simulink model "w2_warplab_trigger_proc"  (Simulink 7.7)
settings: Solver=ode45  StartTime=0.0  StopTime=1000  RelTol=1e-3
InitFcn:
  | w2_warplab_trigger_proc_init
StartFcn:
  | w2_warplab_trigger_proc_init
undefined symbols (not defined in the file or in its folder): gcbh, xlBlockLoadCallback, xlGetNormalizedPeriod
libraries: xbsIndex_r4 x819, simulink x1
(part 6 of 6)

== system w2_warplab_trigger_proc/Trigger Sources/Energy/AntB Detector/Busy Detection ==
  Avg RSSI : Inport
  Reset : Inport  Port=2
  en : Inport  Port=3
  Convert1 : xbsIndex_r4/Convert  gui_display_data_type=Fixed-point  arith_type=Unsigned  n_bits=1  bin_pt=0  float_type=Single  exp_bits=8  fraction_bits=24  quantization=Truncate  overflow=Wrap  en=off  latency=0  dbl_ovrd=off  pipeline=off  block_type=convert
      settings: block_version=VER_STRING_GOES_HERE
  Counter1 : xbsIndex_r4/Counter  cnt_type=Free Running  cnt_to=Inf  operation=Up  start_count=0  cnt_by_val=1  arith_type=Unsigned  n_bits=11  bin_pt=0  load_pin=off  rst=on  en=on  explicit_period=off  period=4  dbl_ovrd=off  use_behavioral_HDL=off  implementation=Fabric  use_rpm=off  block_type=counter
  Inverter1 : xbsIndex_r4/Inverter  en=off  latency=0  dbl_ovrd=off  block_type=inv
      settings: xl_area=[0 0 0 0 0 0 0]  block_version=8.2
  Logical : xbsIndex_r4/Logical  logical_function=AND  inputs=2  en=off  latency=0  precision=Full  arith_type=Unsigned  n_bits=16  bin_pt=0  align_bp=on  dbl_ovrd=off  block_type=logical
  Logical1 : xbsIndex_r4/Logical  logical_function=OR  inputs=2  en=off  latency=0  precision=Full  arith_type=Unsigned  n_bits=16  bin_pt=0  align_bp=on  dbl_ovrd=off  block_type=logical
  Relational2 : xbsIndex_r4/Relational  mode=a>b  en=off  latency=0  dbl_ovrd=off  block_type=relational
      settings: block_version=VER_STRING_GOES_HERE
  Relational3 : xbsIndex_r4/Relational  mode=a>b  en=off  latency=0  dbl_ovrd=off  block_type=relational
      settings: block_version=VER_STRING_GOES_HERE
  S-R Latch : Subsystem
  Busy : Outport
  wires:
  [pktDet_energyThresh_busy] -> Relational2/2
  Reset/1 -> Logical1/1
  Logical1/1 -> Counter1/1, S-R Latch/1(R)
  Inverter1/1 -> Logical1/2
  Counter1/1 -> Relational3/1
  [pktDet_duration_busy] -> Relational3/2
  Relational3/1 -> S-R Latch/2(S)
  S-R Latch/1(Q) -> Convert1/1
  Avg RSSI/1 -> Relational2/1
  Convert1/1 -> Busy/1
  Logical/1 -> Counter1/2
  Relational2/1 -> Logical/1, Inverter1/1
  en/1 -> Logical/2

== system w2_warplab_trigger_proc/Trigger Sources/Energy/AntB Detector/Idle Detection ==
  Avg RSSI : Inport
  Reset : Inport  Port=2
  en : Inport  Port=3
  Convert1 : xbsIndex_r4/Convert  gui_display_data_type=Fixed-point  arith_type=Unsigned  n_bits=1  bin_pt=0  float_type=Single  exp_bits=8  fraction_bits=24  quantization=Truncate  overflow=Wrap  en=off  latency=0  dbl_ovrd=off  pipeline=off  block_type=convert
      settings: block_version=VER_STRING_GOES_HERE
  Counter1 : xbsIndex_r4/Counter  cnt_type=Free Running  cnt_to=Inf  operation=Up  start_count=0  cnt_by_val=1  arith_type=Unsigned  n_bits=11  bin_pt=0  load_pin=off  rst=on  en=on  explicit_period=off  period=4  dbl_ovrd=off  use_behavioral_HDL=off  implementation=Fabric  use_rpm=off  block_type=counter
  Inverter1 : xbsIndex_r4/Inverter  en=off  latency=0  dbl_ovrd=off  block_type=inv
      settings: xl_area=[0 0 0 0 0 0 0]  block_version=8.2
  Logical : xbsIndex_r4/Logical  logical_function=AND  inputs=2  en=off  latency=0  precision=Full  arith_type=Unsigned  n_bits=16  bin_pt=0  align_bp=on  dbl_ovrd=off  block_type=logical
  Logical1 : xbsIndex_r4/Logical  logical_function=OR  inputs=2  en=off  latency=0  precision=Full  arith_type=Unsigned  n_bits=16  bin_pt=0  align_bp=on  dbl_ovrd=off  block_type=logical
  Relational2 : xbsIndex_r4/Relational  mode=a<b  en=off  latency=0  dbl_ovrd=off  block_type=relational
      settings: block_version=VER_STRING_GOES_HERE
  Relational3 : xbsIndex_r4/Relational  mode=a>b  en=off  latency=0  dbl_ovrd=off  block_type=relational
      settings: block_version=VER_STRING_GOES_HERE
  S-R Latch : Subsystem
  Idle : Outport
  wires:
  Convert1/1 -> Idle/1
  Avg RSSI/1 -> Relational2/1
  S-R Latch/1(Q) -> Convert1/1
  Relational3/1 -> S-R Latch/2(S)
  [pktDet_duration_idle] -> Relational3/2
  Counter1/1 -> Relational3/1
  Inverter1/1 -> Logical1/2
  Logical1/1 -> Counter1/1, S-R Latch/1(R)
  Reset/1 -> Logical1/1
  Relational2/1 -> Logical/1, Inverter1/1
  [pktDet_energyThresh_idle] -> Relational2/2
  en/1 -> Logical/2
  Logical/1 -> Counter1/2

== system w2_warplab_trigger_proc/Trigger Sources/Energy/AntB Detector/Running Sum ==
  note: This block impelemnts a variable-length running sum.
      | For a sum y(n) of the previous N samples of sequence x(n), it implements
      | y(n) = y(n-1) + x(n) - x(n-N)
      | This requires a careful reset procedure, where the full shift register
      | is zerored out. Otherwise the feedback-based sum stops working.
  RSSI : Inport
  reset : Inport  Port=2
  avglen : Inport  Port=3
  en : Inport  Port=4
  ASR : xbsIndex_r4/Addressable Shift Register  infer_latency=on  depth=2  initVector=[0]  en=on  dbl_ovrd=off  use_behavioral_HDL=off  Optimization=Resource  use_rpm=off  block_type=addrsr
      settings: infoedit="Delay of configurable length.  Any element in the delay line can be addressed and driven onto the output port.<br><br>Hardware notes: This block is implemented using SRL16s. If Virtex-4 or Spartan-3 device is used, multiple SRLC16s are cascaded together."  block_version=VER_STRING_GOES_HERE
  Accumulator : xbsIndex_r4/Accumulator  operation=Add  n_bits=17  overflow=Flag as error  scale=1  rst=on  infoeditControl=reset for floating point data type must be asserted for a minimum of 2 cycles  hasbypass=off  en=on  latency=0  dbl_ovrd=off  msb_inp=100  msb=100  lsb=-100  use_behavioral_HDL=on  implementation=Fabric  block_type=accum
      settings: block_version=VER_STRING_GOES_HERE
  AddSub : xbsIndex_r4/AddSub  mode=Subtraction  use_carryin=off  use_carryout=off  en=off  latency=0  precision=Full  arith_type=Unsigned  n_bits=10  bin_pt=0  quantization=Truncate  overflow=Wrap  dbl_ovrd=off  use_behavioral_HDL=off  hw_selection=Fabric  pipelined=off  use_rpm=on  block_type=addsub
      settings: block_version=VER_STRING_GOES_HERE
  Convert7 : xbsIndex_r4/Convert  gui_display_data_type=Fixed-point  arith_type=Unsigned  n_bits=17  bin_pt=0  float_type=Single  exp_bits=8  fraction_bits=24  quantization=Truncate  overflow=Saturate  en=off  latency=0  dbl_ovrd=off  pipeline=off  block_type=convert
      settings: block_version=10.1.3
  Logical : xbsIndex_r4/Logical  logical_function=OR  inputs=2  en=off  latency=0  precision=Full  arith_type=Unsigned  n_bits=16  bin_pt=0  align_bp=on  dbl_ovrd=off  block_type=logical
  Long Reset Gen : Subsystem
  Register : xbsIndex_r4/Register  init=0  rst=on  en=off  dbl_ovrd=off  block_type=register
      settings: block_version=VER_STRING_GOES_HERE
  avg : Outport
  wires:
  en/1 -> Accumulator/3, ASR/3
  Convert7/1 -> avg/1
  Long Reset Gen/1(reset_out) -> Logical/1
  reset/1 -> Logical/2, Long Reset Gen/2(reset_in)
  Logical/1 -> Accumulator/2, Register/2
  Accumulator/1 -> Convert7/1
  RSSI/1 -> Register/1
  avglen/1 -> Long Reset Gen/1(duration), ASR/2
  Register/1 -> AddSub/1, ASR/1
  AddSub/1 -> Accumulator/1
  ASR/1 -> AddSub/2

== system w2_warplab_trigger_proc/Trigger Sources/Energy/AntC Detector/Busy Detection ==
  Avg RSSI : Inport
  Reset : Inport  Port=2
  en : Inport  Port=3
  Convert1 : xbsIndex_r4/Convert  gui_display_data_type=Fixed-point  arith_type=Unsigned  n_bits=1  bin_pt=0  float_type=Single  exp_bits=8  fraction_bits=24  quantization=Truncate  overflow=Wrap  en=off  latency=0  dbl_ovrd=off  pipeline=off  block_type=convert
      settings: block_version=VER_STRING_GOES_HERE
  Counter1 : xbsIndex_r4/Counter  cnt_type=Free Running  cnt_to=Inf  operation=Up  start_count=0  cnt_by_val=1  arith_type=Unsigned  n_bits=11  bin_pt=0  load_pin=off  rst=on  en=on  explicit_period=off  period=4  dbl_ovrd=off  use_behavioral_HDL=off  implementation=Fabric  use_rpm=off  block_type=counter
  Inverter1 : xbsIndex_r4/Inverter  en=off  latency=0  dbl_ovrd=off  block_type=inv
      settings: xl_area=[0 0 0 0 0 0 0]  block_version=8.2
  Logical : xbsIndex_r4/Logical  logical_function=AND  inputs=2  en=off  latency=0  precision=Full  arith_type=Unsigned  n_bits=16  bin_pt=0  align_bp=on  dbl_ovrd=off  block_type=logical
  Logical1 : xbsIndex_r4/Logical  logical_function=OR  inputs=2  en=off  latency=0  precision=Full  arith_type=Unsigned  n_bits=16  bin_pt=0  align_bp=on  dbl_ovrd=off  block_type=logical
  Relational2 : xbsIndex_r4/Relational  mode=a>b  en=off  latency=0  dbl_ovrd=off  block_type=relational
      settings: block_version=VER_STRING_GOES_HERE
  Relational3 : xbsIndex_r4/Relational  mode=a>b  en=off  latency=0  dbl_ovrd=off  block_type=relational
      settings: block_version=VER_STRING_GOES_HERE
  S-R Latch : Subsystem
  Busy : Outport
  wires:
  [pktDet_energyThresh_busy] -> Relational2/2
  Reset/1 -> Logical1/1
  Logical1/1 -> Counter1/1, S-R Latch/1(R)
  Inverter1/1 -> Logical1/2
  Counter1/1 -> Relational3/1
  [pktDet_duration_busy] -> Relational3/2
  Relational3/1 -> S-R Latch/2(S)
  S-R Latch/1(Q) -> Convert1/1
  Avg RSSI/1 -> Relational2/1
  Convert1/1 -> Busy/1
  Logical/1 -> Counter1/2
  Relational2/1 -> Logical/1, Inverter1/1
  en/1 -> Logical/2

== system w2_warplab_trigger_proc/Trigger Sources/Energy/AntC Detector/Idle Detection ==
  Avg RSSI : Inport
  Reset : Inport  Port=2
  en : Inport  Port=3
  Convert1 : xbsIndex_r4/Convert  gui_display_data_type=Fixed-point  arith_type=Unsigned  n_bits=1  bin_pt=0  float_type=Single  exp_bits=8  fraction_bits=24  quantization=Truncate  overflow=Wrap  en=off  latency=0  dbl_ovrd=off  pipeline=off  block_type=convert
      settings: block_version=VER_STRING_GOES_HERE
  Counter1 : xbsIndex_r4/Counter  cnt_type=Free Running  cnt_to=Inf  operation=Up  start_count=0  cnt_by_val=1  arith_type=Unsigned  n_bits=11  bin_pt=0  load_pin=off  rst=on  en=on  explicit_period=off  period=4  dbl_ovrd=off  use_behavioral_HDL=off  implementation=Fabric  use_rpm=off  block_type=counter
  Inverter1 : xbsIndex_r4/Inverter  en=off  latency=0  dbl_ovrd=off  block_type=inv
      settings: xl_area=[0 0 0 0 0 0 0]  block_version=8.2
  Logical : xbsIndex_r4/Logical  logical_function=AND  inputs=2  en=off  latency=0  precision=Full  arith_type=Unsigned  n_bits=16  bin_pt=0  align_bp=on  dbl_ovrd=off  block_type=logical
  Logical1 : xbsIndex_r4/Logical  logical_function=OR  inputs=2  en=off  latency=0  precision=Full  arith_type=Unsigned  n_bits=16  bin_pt=0  align_bp=on  dbl_ovrd=off  block_type=logical
  Relational2 : xbsIndex_r4/Relational  mode=a<b  en=off  latency=0  dbl_ovrd=off  block_type=relational
      settings: block_version=VER_STRING_GOES_HERE
  Relational3 : xbsIndex_r4/Relational  mode=a>b  en=off  latency=0  dbl_ovrd=off  block_type=relational
      settings: block_version=VER_STRING_GOES_HERE
  S-R Latch : Subsystem
  Idle : Outport
  wires:
  Convert1/1 -> Idle/1
  Avg RSSI/1 -> Relational2/1
  S-R Latch/1(Q) -> Convert1/1
  Relational3/1 -> S-R Latch/2(S)
  [pktDet_duration_idle] -> Relational3/2
  Counter1/1 -> Relational3/1
  Inverter1/1 -> Logical1/2
  Logical1/1 -> Counter1/1, S-R Latch/1(R)
  Reset/1 -> Logical1/1
  Relational2/1 -> Logical/1, Inverter1/1
  [pktDet_energyThresh_idle] -> Relational2/2
  en/1 -> Logical/2
  Logical/1 -> Counter1/2

== system w2_warplab_trigger_proc/Trigger Sources/Energy/AntC Detector/Running Sum ==
  note: This block impelemnts a variable-length running sum.
      | For a sum y(n) of the previous N samples of sequence x(n), it implements
      | y(n) = y(n-1) + x(n) - x(n-N)
      | This requires a careful reset procedure, where the full shift register
      | is zerored out. Otherwise the feedback-based sum stops working.
  RSSI : Inport
  reset : Inport  Port=2
  avglen : Inport  Port=3
  en : Inport  Port=4
  ASR : xbsIndex_r4/Addressable Shift Register  infer_latency=on  depth=2  initVector=[0]  en=on  dbl_ovrd=off  use_behavioral_HDL=off  Optimization=Resource  use_rpm=off  block_type=addrsr
      settings: infoedit="Delay of configurable length.  Any element in the delay line can be addressed and driven onto the output port.<br><br>Hardware notes: This block is implemented using SRL16s. If Virtex-4 or Spartan-3 device is used, multiple SRLC16s are cascaded together."  block_version=VER_STRING_GOES_HERE
  Accumulator : xbsIndex_r4/Accumulator  operation=Add  n_bits=17  overflow=Flag as error  scale=1  rst=on  infoeditControl=reset for floating point data type must be asserted for a minimum of 2 cycles  hasbypass=off  en=on  latency=0  dbl_ovrd=off  msb_inp=100  msb=100  lsb=-100  use_behavioral_HDL=on  implementation=Fabric  block_type=accum
      settings: block_version=VER_STRING_GOES_HERE
  AddSub : xbsIndex_r4/AddSub  mode=Subtraction  use_carryin=off  use_carryout=off  en=off  latency=0  precision=Full  arith_type=Unsigned  n_bits=10  bin_pt=0  quantization=Truncate  overflow=Wrap  dbl_ovrd=off  use_behavioral_HDL=off  hw_selection=Fabric  pipelined=off  use_rpm=on  block_type=addsub
      settings: block_version=VER_STRING_GOES_HERE
  Convert7 : xbsIndex_r4/Convert  gui_display_data_type=Fixed-point  arith_type=Unsigned  n_bits=17  bin_pt=0  float_type=Single  exp_bits=8  fraction_bits=24  quantization=Truncate  overflow=Saturate  en=off  latency=0  dbl_ovrd=off  pipeline=off  block_type=convert
      settings: block_version=10.1.3
  Logical : xbsIndex_r4/Logical  logical_function=OR  inputs=2  en=off  latency=0  precision=Full  arith_type=Unsigned  n_bits=16  bin_pt=0  align_bp=on  dbl_ovrd=off  block_type=logical
  Long Reset Gen : Subsystem
  Register : xbsIndex_r4/Register  init=0  rst=on  en=off  dbl_ovrd=off  block_type=register
      settings: block_version=VER_STRING_GOES_HERE
  avg : Outport
  wires:
  ASR/1 -> AddSub/2
  AddSub/1 -> Accumulator/1
  Register/1 -> ASR/1, AddSub/1
  avglen/1 -> ASR/2, Long Reset Gen/1(duration)
  RSSI/1 -> Register/1
  Accumulator/1 -> Convert7/1
  Logical/1 -> Register/2, Accumulator/2
  reset/1 -> Long Reset Gen/2(reset_in), Logical/2
  Long Reset Gen/1(reset_out) -> Logical/1
  Convert7/1 -> avg/1
  en/1 -> ASR/3, Accumulator/3

== system w2_warplab_trigger_proc/Trigger Sources/Energy/AntD Detector/Busy Detection ==
  Avg RSSI : Inport
  Reset : Inport  Port=2
  en : Inport  Port=3
  Convert1 : xbsIndex_r4/Convert  gui_display_data_type=Fixed-point  arith_type=Unsigned  n_bits=1  bin_pt=0  float_type=Single  exp_bits=8  fraction_bits=24  quantization=Truncate  overflow=Wrap  en=off  latency=0  dbl_ovrd=off  pipeline=off  block_type=convert
      settings: block_version=VER_STRING_GOES_HERE
  Counter1 : xbsIndex_r4/Counter  cnt_type=Free Running  cnt_to=Inf  operation=Up  start_count=0  cnt_by_val=1  arith_type=Unsigned  n_bits=11  bin_pt=0  load_pin=off  rst=on  en=on  explicit_period=off  period=4  dbl_ovrd=off  use_behavioral_HDL=off  implementation=Fabric  use_rpm=off  block_type=counter
  Inverter1 : xbsIndex_r4/Inverter  en=off  latency=0  dbl_ovrd=off  block_type=inv
      settings: xl_area=[0 0 0 0 0 0 0]  block_version=8.2
  Logical : xbsIndex_r4/Logical  logical_function=AND  inputs=2  en=off  latency=0  precision=Full  arith_type=Unsigned  n_bits=16  bin_pt=0  align_bp=on  dbl_ovrd=off  block_type=logical
  Logical1 : xbsIndex_r4/Logical  logical_function=OR  inputs=2  en=off  latency=0  precision=Full  arith_type=Unsigned  n_bits=16  bin_pt=0  align_bp=on  dbl_ovrd=off  block_type=logical
  Relational2 : xbsIndex_r4/Relational  mode=a>b  en=off  latency=0  dbl_ovrd=off  block_type=relational
      settings: block_version=VER_STRING_GOES_HERE
  Relational3 : xbsIndex_r4/Relational  mode=a>b  en=off  latency=0  dbl_ovrd=off  block_type=relational
      settings: block_version=VER_STRING_GOES_HERE
  S-R Latch : Subsystem
  Busy : Outport
  wires:
  [pktDet_energyThresh_busy] -> Relational2/2
  Reset/1 -> Logical1/1
  Logical1/1 -> Counter1/1, S-R Latch/1(R)
  Inverter1/1 -> Logical1/2
  Counter1/1 -> Relational3/1
  [pktDet_duration_busy] -> Relational3/2
  Relational3/1 -> S-R Latch/2(S)
  S-R Latch/1(Q) -> Convert1/1
  Avg RSSI/1 -> Relational2/1
  Convert1/1 -> Busy/1
  Logical/1 -> Counter1/2
  Relational2/1 -> Logical/1, Inverter1/1
  en/1 -> Logical/2

== system w2_warplab_trigger_proc/Trigger Sources/Energy/AntD Detector/Idle Detection ==
  Avg RSSI : Inport
  Reset : Inport  Port=2
  en : Inport  Port=3
  Convert1 : xbsIndex_r4/Convert  gui_display_data_type=Fixed-point  arith_type=Unsigned  n_bits=1  bin_pt=0  float_type=Single  exp_bits=8  fraction_bits=24  quantization=Truncate  overflow=Wrap  en=off  latency=0  dbl_ovrd=off  pipeline=off  block_type=convert
      settings: block_version=VER_STRING_GOES_HERE
  Counter1 : xbsIndex_r4/Counter  cnt_type=Free Running  cnt_to=Inf  operation=Up  start_count=0  cnt_by_val=1  arith_type=Unsigned  n_bits=11  bin_pt=0  load_pin=off  rst=on  en=on  explicit_period=off  period=4  dbl_ovrd=off  use_behavioral_HDL=off  implementation=Fabric  use_rpm=off  block_type=counter
  Inverter1 : xbsIndex_r4/Inverter  en=off  latency=0  dbl_ovrd=off  block_type=inv
      settings: xl_area=[0 0 0 0 0 0 0]  block_version=8.2
  Logical : xbsIndex_r4/Logical  logical_function=AND  inputs=2  en=off  latency=0  precision=Full  arith_type=Unsigned  n_bits=16  bin_pt=0  align_bp=on  dbl_ovrd=off  block_type=logical
  Logical1 : xbsIndex_r4/Logical  logical_function=OR  inputs=2  en=off  latency=0  precision=Full  arith_type=Unsigned  n_bits=16  bin_pt=0  align_bp=on  dbl_ovrd=off  block_type=logical
  Relational2 : xbsIndex_r4/Relational  mode=a<b  en=off  latency=0  dbl_ovrd=off  block_type=relational
      settings: block_version=VER_STRING_GOES_HERE
  Relational3 : xbsIndex_r4/Relational  mode=a>b  en=off  latency=0  dbl_ovrd=off  block_type=relational
      settings: block_version=VER_STRING_GOES_HERE
  S-R Latch : Subsystem
  Idle : Outport
  wires:
  Convert1/1 -> Idle/1
  Avg RSSI/1 -> Relational2/1
  S-R Latch/1(Q) -> Convert1/1
  Relational3/1 -> S-R Latch/2(S)
  [pktDet_duration_idle] -> Relational3/2
  Counter1/1 -> Relational3/1
  Inverter1/1 -> Logical1/2
  Logical1/1 -> Counter1/1, S-R Latch/1(R)
  Reset/1 -> Logical1/1
  Relational2/1 -> Logical/1, Inverter1/1
  [pktDet_energyThresh_idle] -> Relational2/2
  en/1 -> Logical/2
  Logical/1 -> Counter1/2

== system w2_warplab_trigger_proc/Trigger Sources/Energy/AntD Detector/Running Sum ==
  note: This block impelemnts a variable-length running sum.
      | For a sum y(n) of the previous N samples of sequence x(n), it implements
      | y(n) = y(n-1) + x(n) - x(n-N)
      | This requires a careful reset procedure, where the full shift register
      | is zerored out. Otherwise the feedback-based sum stops working.
  RSSI : Inport
  reset : Inport  Port=2
  avglen : Inport  Port=3
  en : Inport  Port=4
  ASR : xbsIndex_r4/Addressable Shift Register  infer_latency=on  depth=2  initVector=[0]  en=on  dbl_ovrd=off  use_behavioral_HDL=off  Optimization=Resource  use_rpm=off  block_type=addrsr
      settings: infoedit="Delay of configurable length.  Any element in the delay line can be addressed and driven onto the output port.<br><br>Hardware notes: This block is implemented using SRL16s. If Virtex-4 or Spartan-3 device is used, multiple SRLC16s are cascaded together."  block_version=VER_STRING_GOES_HERE
  Accumulator : xbsIndex_r4/Accumulator  operation=Add  n_bits=17  overflow=Flag as error  scale=1  rst=on  infoeditControl=reset for floating point data type must be asserted for a minimum of 2 cycles  hasbypass=off  en=on  latency=0  dbl_ovrd=off  msb_inp=100  msb=100  lsb=-100  use_behavioral_HDL=on  implementation=Fabric  block_type=accum
      settings: block_version=VER_STRING_GOES_HERE
  AddSub : xbsIndex_r4/AddSub  mode=Subtraction  use_carryin=off  use_carryout=off  en=off  latency=0  precision=Full  arith_type=Unsigned  n_bits=10  bin_pt=0  quantization=Truncate  overflow=Wrap  dbl_ovrd=off  use_behavioral_HDL=off  hw_selection=Fabric  pipelined=off  use_rpm=on  block_type=addsub
      settings: block_version=VER_STRING_GOES_HERE
  Convert7 : xbsIndex_r4/Convert  gui_display_data_type=Fixed-point  arith_type=Unsigned  n_bits=17  bin_pt=0  float_type=Single  exp_bits=8  fraction_bits=24  quantization=Truncate  overflow=Saturate  en=off  latency=0  dbl_ovrd=off  pipeline=off  block_type=convert
      settings: block_version=10.1.3
  Logical : xbsIndex_r4/Logical  logical_function=OR  inputs=2  en=off  latency=0  precision=Full  arith_type=Unsigned  n_bits=16  bin_pt=0  align_bp=on  dbl_ovrd=off  block_type=logical
  Long Reset Gen : Subsystem
  Register : xbsIndex_r4/Register  init=0  rst=on  en=off  dbl_ovrd=off  block_type=register
      settings: block_version=VER_STRING_GOES_HERE
  avg : Outport
  wires:
  en/1 -> Accumulator/3, ASR/3
  Convert7/1 -> avg/1
  Long Reset Gen/1(reset_out) -> Logical/1
  reset/1 -> Logical/2, Long Reset Gen/2(reset_in)
  Logical/1 -> Accumulator/2, Register/2
  Accumulator/1 -> Convert7/1
  RSSI/1 -> Register/1
  avglen/1 -> Long Reset Gen/1(duration), ASR/2
  Register/1 -> AddSub/1, ASR/1
  AddSub/1 -> Accumulator/1
  ASR/1 -> AddSub/2

== system w2_warplab_trigger_proc/Trigger Sources/Energy/AntA Detector/Busy Detection/S-R Latch ==
  R : Inport
  S : Inport  Port=2
  Constant1 : xbsIndex_r4/Constant  const=1  gui_display_data_type=Fixed-point  arith_type=Boolean  n_bits=1  bin_pt=0  preci_type=Single  exp_width=8  frac_width=24  explicit_period=off  period=1  equ=P=C  opselect=C  inp2=PCIN>>17  opr=+  inp1=P  carry=CIN  dbl_ovrd=off  block_type=constant
      settings: block_version=VER_STRING_GOES_HERE
  Register2 : xbsIndex_r4/Register  init=0  rst=on  en=on  dbl_ovrd=off  block_type=register
      settings: xl_area=[1 1 0 0 0 0 0]  block_version=VER_STRING_GOES_HERE
  Q : Outport
  wires:
  Constant1/1 -> Register2/1
  R/1 -> Register2/2
  Register2/1 -> Q/1
  S/1 -> Register2/3

== system w2_warplab_trigger_proc/Trigger Sources/Energy/AntA Detector/Idle Detection/S-R Latch ==
  R : Inport
  S : Inport  Port=2
  Constant1 : xbsIndex_r4/Constant  const=1  gui_display_data_type=Fixed-point  arith_type=Boolean  n_bits=1  bin_pt=0  preci_type=Single  exp_width=8  frac_width=24  explicit_period=off  period=1  equ=P=C  opselect=C  inp2=PCIN>>17  opr=+  inp1=P  carry=CIN  dbl_ovrd=off  block_type=constant
      settings: block_version=VER_STRING_GOES_HERE
  Register2 : xbsIndex_r4/Register  init=0  rst=on  en=on  dbl_ovrd=off  block_type=register
      settings: xl_area=[1 1 0 0 0 0 0]  block_version=VER_STRING_GOES_HERE
  Q : Outport
  wires:
  S/1 -> Register2/3
  Register2/1 -> Q/1
  R/1 -> Register2/2
  Constant1/1 -> Register2/1

== system w2_warplab_trigger_proc/Trigger Sources/Energy/AntA Detector/Running Sum/Long Reset Gen ==
  duration : Inport
  reset_in : Inport  Port=2
  Counter : xbsIndex_r4/Counter  cnt_type=Free Running  cnt_to=0  operation=Up  start_count=0  cnt_by_val=1  arith_type=Unsigned  n_bits=8  bin_pt=0  load_pin=off  rst=on  en=on  explicit_period=off  period=4  dbl_ovrd=off  use_behavioral_HDL=off  implementation=Fabric  use_rpm=off  block_type=counter
      settings: block_version=VER_STRING_GOES_HERE
  Relational : xbsIndex_r4/Relational  mode=a=b  en=off  latency=0  dbl_ovrd=off  block_type=relational
      settings: block_version=VER_STRING_GOES_HERE
  S-R Latch : Subsystem
  reset_out : Outport
  wires:
  Relational/1 -> Counter/1, S-R Latch/2(R)
  Counter/1 -> Relational/1
  reset_in/1 -> S-R Latch/1(S)
  duration/1 -> Relational/2
  S-R Latch/1(Q) -> Counter/2, reset_out/1

== system w2_warplab_trigger_proc/Trigger Sources/Energy/AntB Detector/Busy Detection/S-R Latch ==
  R : Inport
  S : Inport  Port=2
  Constant1 : xbsIndex_r4/Constant  const=1  gui_display_data_type=Fixed-point  arith_type=Boolean  n_bits=1  bin_pt=0  preci_type=Single  exp_width=8  frac_width=24  explicit_period=off  period=1  equ=P=C  opselect=C  inp2=PCIN>>17  opr=+  inp1=P  carry=CIN  dbl_ovrd=off  block_type=constant
      settings: block_version=VER_STRING_GOES_HERE
  Register2 : xbsIndex_r4/Register  init=0  rst=on  en=on  dbl_ovrd=off  block_type=register
      settings: xl_area=[1 1 0 0 0 0 0]  block_version=VER_STRING_GOES_HERE
  Q : Outport
  wires:
  Constant1/1 -> Register2/1
  R/1 -> Register2/2
  Register2/1 -> Q/1
  S/1 -> Register2/3

== system w2_warplab_trigger_proc/Trigger Sources/Energy/AntB Detector/Idle Detection/S-R Latch ==
  R : Inport
  S : Inport  Port=2
  Constant1 : xbsIndex_r4/Constant  const=1  gui_display_data_type=Fixed-point  arith_type=Boolean  n_bits=1  bin_pt=0  preci_type=Single  exp_width=8  frac_width=24  explicit_period=off  period=1  equ=P=C  opselect=C  inp2=PCIN>>17  opr=+  inp1=P  carry=CIN  dbl_ovrd=off  block_type=constant
      settings: block_version=VER_STRING_GOES_HERE
  Register2 : xbsIndex_r4/Register  init=0  rst=on  en=on  dbl_ovrd=off  block_type=register
      settings: xl_area=[1 1 0 0 0 0 0]  block_version=VER_STRING_GOES_HERE
  Q : Outport
  wires:
  S/1 -> Register2/3
  Register2/1 -> Q/1
  R/1 -> Register2/2
  Constant1/1 -> Register2/1

== system w2_warplab_trigger_proc/Trigger Sources/Energy/AntB Detector/Running Sum/Long Reset Gen ==
  duration : Inport
  reset_in : Inport  Port=2
  Counter : xbsIndex_r4/Counter  cnt_type=Free Running  cnt_to=0  operation=Up  start_count=0  cnt_by_val=1  arith_type=Unsigned  n_bits=8  bin_pt=0  load_pin=off  rst=on  en=on  explicit_period=off  period=4  dbl_ovrd=off  use_behavioral_HDL=off  implementation=Fabric  use_rpm=off  block_type=counter
      settings: block_version=VER_STRING_GOES_HERE
  Relational : xbsIndex_r4/Relational  mode=a=b  en=off  latency=0  dbl_ovrd=off  block_type=relational
      settings: block_version=VER_STRING_GOES_HERE
  S-R Latch : Subsystem
  reset_out : Outport
  wires:
  S-R Latch/1(Q) -> reset_out/1, Counter/2
  duration/1 -> Relational/2
  reset_in/1 -> S-R Latch/1(S)
  Counter/1 -> Relational/1
  Relational/1 -> S-R Latch/2(R), Counter/1

== system w2_warplab_trigger_proc/Trigger Sources/Energy/AntC Detector/Busy Detection/S-R Latch ==
  R : Inport
  S : Inport  Port=2
  Constant1 : xbsIndex_r4/Constant  const=1  gui_display_data_type=Fixed-point  arith_type=Boolean  n_bits=1  bin_pt=0  preci_type=Single  exp_width=8  frac_width=24  explicit_period=off  period=1  equ=P=C  opselect=C  inp2=PCIN>>17  opr=+  inp1=P  carry=CIN  dbl_ovrd=off  block_type=constant
      settings: block_version=VER_STRING_GOES_HERE
  Register2 : xbsIndex_r4/Register  init=0  rst=on  en=on  dbl_ovrd=off  block_type=register
      settings: xl_area=[1 1 0 0 0 0 0]  block_version=VER_STRING_GOES_HERE
  Q : Outport
  wires:
  Constant1/1 -> Register2/1
  R/1 -> Register2/2
  Register2/1 -> Q/1
  S/1 -> Register2/3

== system w2_warplab_trigger_proc/Trigger Sources/Energy/AntC Detector/Idle Detection/S-R Latch ==
  R : Inport
  S : Inport  Port=2
  Constant1 : xbsIndex_r4/Constant  const=1  gui_display_data_type=Fixed-point  arith_type=Boolean  n_bits=1  bin_pt=0  preci_type=Single  exp_width=8  frac_width=24  explicit_period=off  period=1  equ=P=C  opselect=C  inp2=PCIN>>17  opr=+  inp1=P  carry=CIN  dbl_ovrd=off  block_type=constant
      settings: block_version=VER_STRING_GOES_HERE
  Register2 : xbsIndex_r4/Register  init=0  rst=on  en=on  dbl_ovrd=off  block_type=register
      settings: xl_area=[1 1 0 0 0 0 0]  block_version=VER_STRING_GOES_HERE
  Q : Outport
  wires:
  S/1 -> Register2/3
  Register2/1 -> Q/1
  R/1 -> Register2/2
  Constant1/1 -> Register2/1

== system w2_warplab_trigger_proc/Trigger Sources/Energy/AntC Detector/Running Sum/Long Reset Gen ==
  duration : Inport
  reset_in : Inport  Port=2
  Counter : xbsIndex_r4/Counter  cnt_type=Free Running  cnt_to=0  operation=Up  start_count=0  cnt_by_val=1  arith_type=Unsigned  n_bits=8  bin_pt=0  load_pin=off  rst=on  en=on  explicit_period=off  period=4  dbl_ovrd=off  use_behavioral_HDL=off  implementation=Fabric  use_rpm=off  block_type=counter
      settings: block_version=VER_STRING_GOES_HERE
  Relational : xbsIndex_r4/Relational  mode=a=b  en=off  latency=0  dbl_ovrd=off  block_type=relational
      settings: block_version=VER_STRING_GOES_HERE
  S-R Latch : Subsystem
  reset_out : Outport
  wires:
  Relational/1 -> Counter/1, S-R Latch/2(R)
  Counter/1 -> Relational/1
  reset_in/1 -> S-R Latch/1(S)
  duration/1 -> Relational/2
  S-R Latch/1(Q) -> Counter/2, reset_out/1

== system w2_warplab_trigger_proc/Trigger Sources/Energy/AntD Detector/Busy Detection/S-R Latch ==
  R : Inport
  S : Inport  Port=2
  Constant1 : xbsIndex_r4/Constant  const=1  gui_display_data_type=Fixed-point  arith_type=Boolean  n_bits=1  bin_pt=0  preci_type=Single  exp_width=8  frac_width=24  explicit_period=off  period=1  equ=P=C  opselect=C  inp2=PCIN>>17  opr=+  inp1=P  carry=CIN  dbl_ovrd=off  block_type=constant
      settings: block_version=VER_STRING_GOES_HERE
  Register2 : xbsIndex_r4/Register  init=0  rst=on  en=on  dbl_ovrd=off  block_type=register
      settings: xl_area=[1 1 0 0 0 0 0]  block_version=VER_STRING_GOES_HERE
  Q : Outport
  wires:
  Constant1/1 -> Register2/1
  R/1 -> Register2/2
  Register2/1 -> Q/1
  S/1 -> Register2/3

== system w2_warplab_trigger_proc/Trigger Sources/Energy/AntD Detector/Idle Detection/S-R Latch ==
  R : Inport
  S : Inport  Port=2
  Constant1 : xbsIndex_r4/Constant  const=1  gui_display_data_type=Fixed-point  arith_type=Boolean  n_bits=1  bin_pt=0  preci_type=Single  exp_width=8  frac_width=24  explicit_period=off  period=1  equ=P=C  opselect=C  inp2=PCIN>>17  opr=+  inp1=P  carry=CIN  dbl_ovrd=off  block_type=constant
      settings: block_version=VER_STRING_GOES_HERE
  Register2 : xbsIndex_r4/Register  init=0  rst=on  en=on  dbl_ovrd=off  block_type=register
      settings: xl_area=[1 1 0 0 0 0 0]  block_version=VER_STRING_GOES_HERE
  Q : Outport
  wires:
  S/1 -> Register2/3
  Register2/1 -> Q/1
  R/1 -> Register2/2
  Constant1/1 -> Register2/1

== system w2_warplab_trigger_proc/Trigger Sources/Energy/AntD Detector/Running Sum/Long Reset Gen ==
  duration : Inport
  reset_in : Inport  Port=2
  Counter : xbsIndex_r4/Counter  cnt_type=Free Running  cnt_to=0  operation=Up  start_count=0  cnt_by_val=1  arith_type=Unsigned  n_bits=8  bin_pt=0  load_pin=off  rst=on  en=on  explicit_period=off  period=4  dbl_ovrd=off  use_behavioral_HDL=off  implementation=Fabric  use_rpm=off  block_type=counter
      settings: block_version=VER_STRING_GOES_HERE
  Relational : xbsIndex_r4/Relational  mode=a=b  en=off  latency=0  dbl_ovrd=off  block_type=relational
      settings: block_version=VER_STRING_GOES_HERE
  S-R Latch : Subsystem
  reset_out : Outport
  wires:
  S-R Latch/1(Q) -> reset_out/1, Counter/2
  duration/1 -> Relational/2
  reset_in/1 -> S-R Latch/1(S)
  Counter/1 -> Relational/1
  Relational/1 -> S-R Latch/2(R), Counter/1

== system w2_warplab_trigger_proc/Trigger Sources/Energy/AntA Detector/Running Sum/Long Reset Gen/S-R Latch ==
  S : Inport
  R : Inport  Port=2
  Constant1 : xbsIndex_r4/Constant  const=1  gui_display_data_type=Fixed-point  arith_type=Boolean  n_bits=1  bin_pt=0  preci_type=Single  exp_width=8  frac_width=24  explicit_period=off  period=1  equ=P=C  opselect=C  inp2=PCIN>>17  opr=+  inp1=P  carry=CIN  dbl_ovrd=off  block_type=constant
      settings: block_version=VER_STRING_GOES_HERE
  Register2 : xbsIndex_r4/Register  init=0  rst=on  en=on  dbl_ovrd=off  block_type=register
      settings: xl_area=[1 1 0 0 0 0 0]  block_version=VER_STRING_GOES_HERE
  Q : Outport
  wires:
  Constant1/1 -> Register2/1
  R/1 -> Register2/2
  Register2/1 -> Q/1
  S/1 -> Register2/3

== system w2_warplab_trigger_proc/Trigger Sources/Energy/AntB Detector/Running Sum/Long Reset Gen/S-R Latch ==
  S : Inport
  R : Inport  Port=2
  Constant1 : xbsIndex_r4/Constant  const=1  gui_display_data_type=Fixed-point  arith_type=Boolean  n_bits=1  bin_pt=0  preci_type=Single  exp_width=8  frac_width=24  explicit_period=off  period=1  equ=P=C  opselect=C  inp2=PCIN>>17  opr=+  inp1=P  carry=CIN  dbl_ovrd=off  block_type=constant
      settings: block_version=VER_STRING_GOES_HERE
  Register2 : xbsIndex_r4/Register  init=0  rst=on  en=on  dbl_ovrd=off  block_type=register
      settings: xl_area=[1 1 0 0 0 0 0]  block_version=VER_STRING_GOES_HERE
  Q : Outport
  wires:
  S/1 -> Register2/3
  Register2/1 -> Q/1
  R/1 -> Register2/2
  Constant1/1 -> Register2/1

== system w2_warplab_trigger_proc/Trigger Sources/Energy/AntC Detector/Running Sum/Long Reset Gen/S-R Latch ==
  S : Inport
  R : Inport  Port=2
  Constant1 : xbsIndex_r4/Constant  const=1  gui_display_data_type=Fixed-point  arith_type=Boolean  n_bits=1  bin_pt=0  preci_type=Single  exp_width=8  frac_width=24  explicit_period=off  period=1  equ=P=C  opselect=C  inp2=PCIN>>17  opr=+  inp1=P  carry=CIN  dbl_ovrd=off  block_type=constant
      settings: block_version=VER_STRING_GOES_HERE
  Register2 : xbsIndex_r4/Register  init=0  rst=on  en=on  dbl_ovrd=off  block_type=register
      settings: xl_area=[1 1 0 0 0 0 0]  block_version=VER_STRING_GOES_HERE
  Q : Outport
  wires:
  Constant1/1 -> Register2/1
  R/1 -> Register2/2
  Register2/1 -> Q/1
  S/1 -> Register2/3

== system w2_warplab_trigger_proc/Trigger Sources/Energy/AntD Detector/Running Sum/Long Reset Gen/S-R Latch ==
  S : Inport
  R : Inport  Port=2
  Constant1 : xbsIndex_r4/Constant  const=1  gui_display_data_type=Fixed-point  arith_type=Boolean  n_bits=1  bin_pt=0  preci_type=Single  exp_width=8  frac_width=24  explicit_period=off  period=1  equ=P=C  opselect=C  inp2=PCIN>>17  opr=+  inp1=P  carry=CIN  dbl_ovrd=off  block_type=constant
      settings: block_version=VER_STRING_GOES_HERE
  Register2 : xbsIndex_r4/Register  init=0  rst=on  en=on  dbl_ovrd=off  block_type=register
      settings: xl_area=[1 1 0 0 0 0 0]  block_version=VER_STRING_GOES_HERE
  Q : Outport
  wires:
  S/1 -> Register2/3
  Register2/1 -> Q/1
  R/1 -> Register2/2
  Constant1/1 -> Register2/1
